simulink model "V605_mathematicalMotorModel"  (R2025a)
settings: Solver=VariableStepAuto  StartTime=0.0  StopTime=10.0  RelTol=1e-3
undefined symbols (not defined in the file or in its folder): prop, rad, s
libraries: aerolibconvert2 x1
settings Model: Creator=Ayush_S  LastModifiedBy=Ayush_S

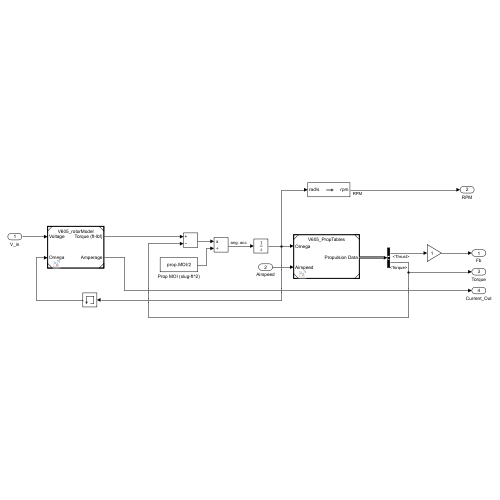
[thumbnail: Simulink's stored preview of the top-level diagram]
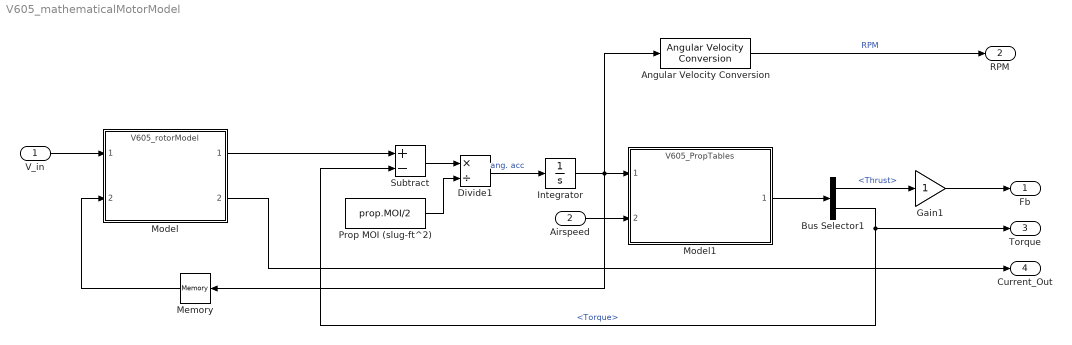
== system V605_mathematicalMotorModel ==
  V_in : Inport
  Airspeed : Inport  Port=2
  Angular Velocity Conversion : aerolibconvert2/Angular Velocity Conversion  IU=rad/s  OU=rpm
  Bus Selector1 : BusSelector  OutputSignals=Thrust,Torque
  Divide1 : Product  Inputs=*/
  Gain1 : Gain
  Integrator : Integrator
  Memory : Memory  InitialCondition=50
  Model : ModelReference  ModelNameDialog=V605_rotorModel.slx  SimulationMode=Normal  ModelReferenceVersion=1.8
  Model1 : ModelReference  ModelNameDialog=V605_PropTables.slx  SimulationMode=Normal  ModelReferenceVersion=1.5
  Prop MOI (slug-ft^2) : Constant  Value=prop.MOI/2
  Subtract : Sum  Inputs=+-
  Fb : Outport
  RPM : Outport  Port=2
  Torque : Outport  Port=3
  Current_Out : Outport  Port=4
  wires:
  Bus Selector1/1 -> Gain1/1  "<Thrust>"
  Subtract/1 -> Divide1/1
  Divide1/1 -> Integrator/1  "ang. acc"
  Bus Selector1/2 -> Subtract/2, Torque/1  "<Torque>"
  Prop MOI (slug-ft^2)/1 -> Divide1/2
  Model1/1 -> Bus Selector1/1
  Model/2 -> Current_Out/1
  Gain1/1 -> Fb/1
  Airspeed/1 -> Model1/2
  V_in/1 -> Model/1
  Angular Velocity Conversion/1 -> RPM/1  "RPM"
  Model/1 -> Subtract/1
  Integrator/1 -> Memory/1, Model1/1, Angular Velocity Conversion/1
  Memory/1 -> Model/2
